simulink model "TestTriggeredSubSystem"  (R2022b)
settings: Solver=VariableStepAuto  StartTime=0.0  StopTime=inf  RelTol=1e-3
model workspace (MAT data in the model file):
  filename = 0
settings Model: Creator=bryantboatright  LastModifiedBy=bryantboatright

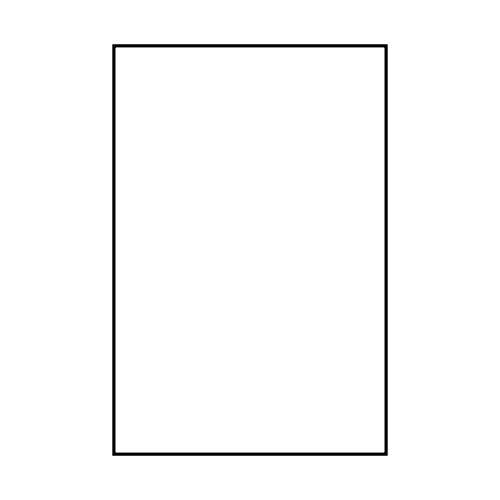
[thumbnail: Simulink's stored preview of the top-level diagram]
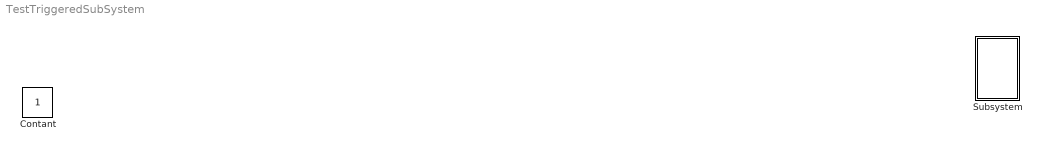
== system TestTriggeredSubSystem ==
  Subsystem : Subsystem
  Contant : Constant  IOType=siggen

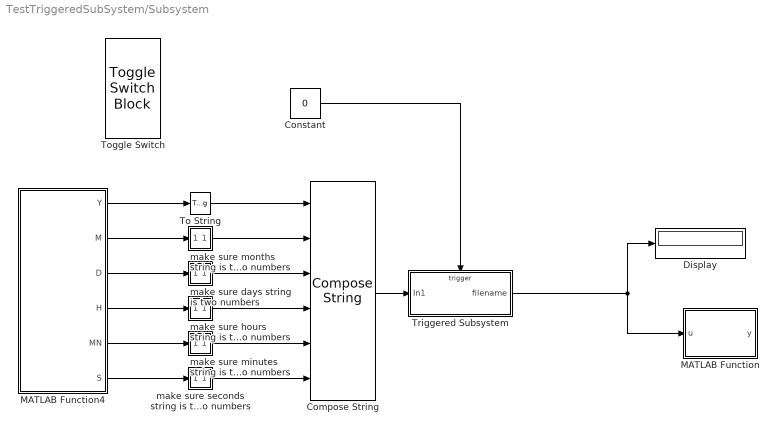
== system TestTriggeredSubSystem/Subsystem ==
  Compose String : ComposeString  Format="\"%s-%s-%s--%s-%s-%s--output.csv\""
  Constant : Constant  Value=0
  Display : Display
  MATLAB Function : MATLAB Function  TreatAsAtomicUnit=on
  MATLAB Function4 : MATLAB Function  TreatAsAtomicUnit=on  SystemSampleTime=200
  To String : ToString
  Toggle Switch : ToggleSwitchBlock
      settings: Values={{'Off', 'On'}, [0 1]}
  Triggered Subsystem : Subsystem  TreatAsAtomicUnit=on
  make sure days string is two numbers : Subsystem
  make sure hours string is two numbers : Subsystem
  make sure minutes string is two numbers : Subsystem
  make sure months string is two numbers : Subsystem
  make sure seconds string is two numbers : Subsystem
  wires:
  make sure seconds string is two numbers/1(Out1) -> Compose String/6
  MATLAB Function4/1(Y) -> To String/1
  MATLAB Function4/3(D) -> make sure days string is two numbers/1(In1)
  Triggered Subsystem/1(filename) -> MATLAB Function/1(u), Display/1
  MATLAB Function4/2(M) -> make sure months string is two numbers/1(In1)
  Constant/1 -> Triggered Subsystem/Trigger
  make sure hours string is two numbers/1(Out1) -> Compose String/4
  MATLAB Function4/4(H) -> make sure hours string is two numbers/1(In1)
  make sure minutes string is two numbers/1(Out1) -> Compose String/5
  make sure days string is two numbers/1(Out1) -> Compose String/3
  MATLAB Function4/5(MN) -> make sure minutes string is two numbers/1(In1)
  Compose String/1 -> Triggered Subsystem/1(In1)
  MATLAB Function4/6(S) -> make sure seconds string is two numbers/1(In1)
  To String/1 -> Compose String/1
  make sure months string is two numbers/1(Out1) -> Compose String/2

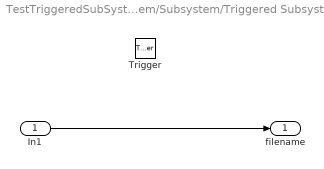
== system TestTriggeredSubSystem/Subsystem/Triggered Subsystem ==
  In1 : Inport
  Trigger : TriggerPort  VariantControl=(inherit)
  filename : Outport
  wires:
  In1/1 -> filename/1

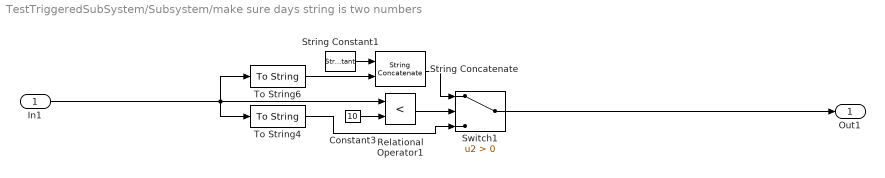
== system TestTriggeredSubSystem/Subsystem/make sure days string is two numbers ==
  In1 : Inport
  Constant3 : Constant  Value=10  VectorParams1D=off  OutDataTypeStr=int8
  Relational Operator1 : RelationalOperator  Operator=<  OutDataTypeStr=boolean  RndMeth=Simplest  InputSameDT=off
  String Concatenate : StringConcatenate
  String Constant1 : StringConstant  String="\"0\""
  Switch1 : Switch  Criteria=u2 > Threshold  SaturateOnIntegerOverflow=off  InputSameDT=off
  To String4 : ToString
  To String6 : ToString
  Out1 : Outport
  wires:
  Constant3/1 -> Relational Operator1/2
  Relational Operator1/1 -> Switch1/2
  To String4/1 -> Switch1/3
  To String6/1 -> String Concatenate/2
  String Constant1/1 -> String Concatenate/1
  String Concatenate/1 -> Switch1/1
  In1/1 -> Relational Operator1/1, To String4/1, To String6/1
  Switch1/1 -> Out1/1

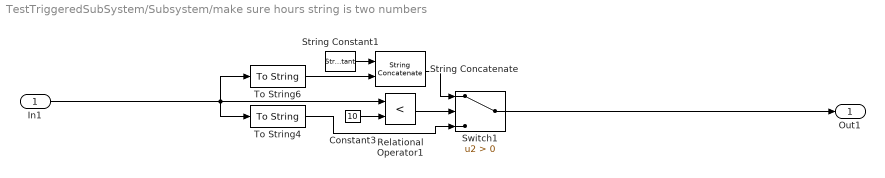
== system TestTriggeredSubSystem/Subsystem/make sure hours string is two numbers ==
  In1 : Inport
  Constant3 : Constant  Value=10  VectorParams1D=off  OutDataTypeStr=int8
  Relational Operator1 : RelationalOperator  Operator=<  OutDataTypeStr=boolean  RndMeth=Simplest  InputSameDT=off
  String Concatenate : StringConcatenate
  String Constant1 : StringConstant  String="\"0\""
  Switch1 : Switch  Criteria=u2 > Threshold  SaturateOnIntegerOverflow=off  InputSameDT=off
  To String4 : ToString
  To String6 : ToString
  Out1 : Outport
  wires:
  Switch1/1 -> Out1/1
  In1/1 -> To String6/1, To String4/1, Relational Operator1/1
  String Concatenate/1 -> Switch1/1
  String Constant1/1 -> String Concatenate/1
  To String6/1 -> String Concatenate/2
  To String4/1 -> Switch1/3
  Relational Operator1/1 -> Switch1/2
  Constant3/1 -> Relational Operator1/2

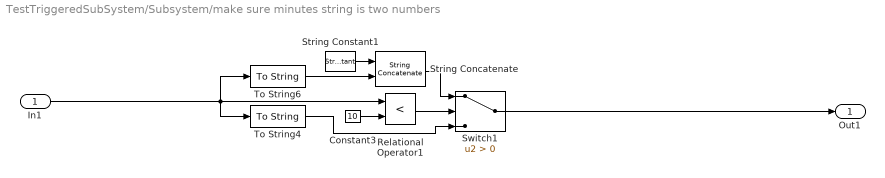
== system TestTriggeredSubSystem/Subsystem/make sure minutes string is two numbers ==
  In1 : Inport
  Constant3 : Constant  Value=10  VectorParams1D=off  OutDataTypeStr=int8
  Relational Operator1 : RelationalOperator  Operator=<  OutDataTypeStr=boolean  RndMeth=Simplest  InputSameDT=off
  String Concatenate : StringConcatenate
  String Constant1 : StringConstant  String="\"0\""
  Switch1 : Switch  Criteria=u2 > Threshold  SaturateOnIntegerOverflow=off  InputSameDT=off
  To String4 : ToString
  To String6 : ToString
  Out1 : Outport
  wires:
  Constant3/1 -> Relational Operator1/2
  Relational Operator1/1 -> Switch1/2
  To String4/1 -> Switch1/3
  To String6/1 -> String Concatenate/2
  String Constant1/1 -> String Concatenate/1
  String Concatenate/1 -> Switch1/1
  In1/1 -> Relational Operator1/1, To String4/1, To String6/1
  Switch1/1 -> Out1/1

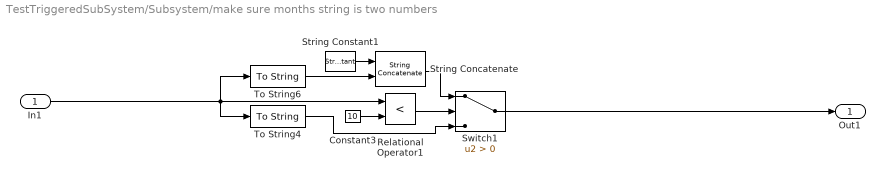
== system TestTriggeredSubSystem/Subsystem/make sure months string is two numbers ==
  In1 : Inport
  Constant3 : Constant  Value=10  VectorParams1D=off  OutDataTypeStr=int8
  Relational Operator1 : RelationalOperator  Operator=<  OutDataTypeStr=boolean  RndMeth=Simplest  InputSameDT=off
  String Concatenate : StringConcatenate
  String Constant1 : StringConstant  String="\"0\""
  Switch1 : Switch  Criteria=u2 > Threshold  SaturateOnIntegerOverflow=off  InputSameDT=off
  To String4 : ToString
  To String6 : ToString
  Out1 : Outport
  wires:
  Switch1/1 -> Out1/1
  In1/1 -> To String6/1, To String4/1, Relational Operator1/1
  String Concatenate/1 -> Switch1/1
  String Constant1/1 -> String Concatenate/1
  To String6/1 -> String Concatenate/2
  To String4/1 -> Switch1/3
  Relational Operator1/1 -> Switch1/2
  Constant3/1 -> Relational Operator1/2

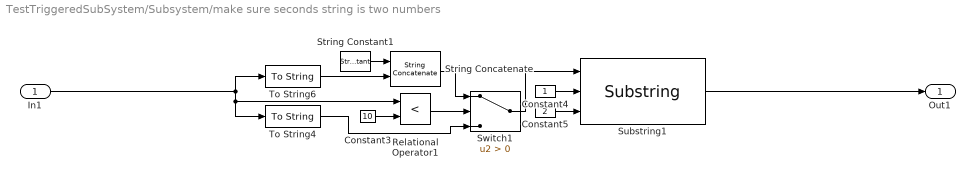
== system TestTriggeredSubSystem/Subsystem/make sure seconds string is two numbers ==
  In1 : Inport
  Constant3 : Constant  Value=10  VectorParams1D=off  OutDataTypeStr=int8
  Constant4 : Constant  VectorParams1D=off  OutDataTypeStr=int8
  Constant5 : Constant  Value=2  VectorParams1D=off  OutDataTypeStr=uint8
  Relational Operator1 : RelationalOperator  Operator=<  OutDataTypeStr=boolean  RndMeth=Simplest  InputSameDT=off
  String Concatenate : StringConcatenate
  String Constant1 : StringConstant  String="\"0\""
  Substring1 : Substring
  Switch1 : Switch  Criteria=u2 > Threshold  SaturateOnIntegerOverflow=off  InputSameDT=off
  To String4 : ToString
  To String6 : ToString
  Out1 : Outport
  wires:
  Substring1/1 -> Out1/1
  To String4/1 -> Switch1/3
  Switch1/1 -> Substring1/1
  Constant3/1 -> Relational Operator1/2
  Constant5/1 -> Substring1/3
  In1/1 -> Relational Operator1/1, To String4/1, To String6/1
  Constant4/1 -> Substring1/2
  Relational Operator1/1 -> Switch1/2
  To String6/1 -> String Concatenate/2
  String Constant1/1 -> String Concatenate/1
  String Concatenate/1 -> Switch1/1

== matlab function TestTriggeredSubSystem/Subsystem/MATLAB Function ==
  data: u input; y output
function y = fcn(u)

if ("" ~= u)
    y =1;
else
    y = -1;
end

== matlab function TestTriggeredSubSystem/Subsystem/MATLAB Function4 ==
  data: Y output; M output; D output; H output; MN output; S output
function [Y, M, D, H, MN, S] = dateGenerator()
   coder.extrinsic('now');
   coder.extrinsic('datevec');
   Y = 0;
   M = 0;
   D = 0;
   H = 0;
   MN = 0;
   S = 0;
   [Y, M, D, H, MN, S] = datevec(datetime("now"));
end
